simulink model "adip_saturation_sim"  (R2013a)
settings: Solver=ode4  StartTime=0.0  StopTime=10  FixedStep=0.001  RelTol=1e-3
values from neighbouring files (symbols this model uses):
  a1 = vertex(1,i)    [p2c13_ex5_adip_lqr_servo.m]    (also in p2c13_ex5_adip_oc_nominal_servo.m; p2c13_ex5_adip_oc_robust_servo.m)
  b1 = vertex(2,i)    [p2c13_ex5_adip_lqr_servo.m]    (also in p2c13_ex5_adip_oc_nominal_servo.m; p2c13_ex5_adip_oc_robust_servo.m)
  dtheta1_0 = 0    [p2c122_ex4_adip_oc_multiobjective_servo.m]    (also in p2c122_ex4_adip_oc_servo.m; p2c13_ex5_adip_lqr_servo.m; p2c13_ex5_adip_oc_nominal_servo.m; p2c13_ex5_adip_oc_robust_servo.m)
  dtheta2_0 = 0    [p2c122_ex4_adip_oc_multiobjective_servo.m]    (also in p2c122_ex4_adip_oc_servo.m; p2c13_ex5_adip_lqr_servo.m; p2c13_ex5_adip_oc_nominal_servo.m; p2c13_ex5_adip_oc_robust_servo.m)
  K = L*inv(X)    [p2c14_ex6_adip_oc_saturation.m]    (also in p2c15_ex7_adip_oc_gs_servo.m; p2c15_ex7_adip_oc_gs_servo_old.m)
  sat = sqrt(sigma2)    [p2c14_ex6_adip_oc_saturation.m]
  theta1_0 = 0    [p2c122_ex4_adip_oc_multiobjective_servo.m]    (also in p2c122_ex4_adip_oc_servo.m; p2c13_ex5_adip_lqr_servo.m; p2c13_ex5_adip_oc_nominal_servo.m; p2c13_ex5_adip_oc_robust_servo.m)
  theta2_0 = 0    [p2c122_ex4_adip_oc_multiobjective_servo.m]    (also in p2c122_ex4_adip_oc_servo.m; p2c13_ex5_adip_lqr_servo.m; p2c13_ex5_adip_oc_nominal_servo.m; p2c13_ex5_adip_oc_robust_servo.m)
undefined symbols (not defined in the file or in its folder): alpha2, alpha3, alpha5, mu2
settings Model: Creator=kawata  LastModifiedBy=kawata
settings DataIOCC: LimitDataPoints=off  SignalLoggingSaveFormat=ModelDataLogs
settings OptimizationCC: ExpressionDepthLimit=2147483647
settings DebuggingCC: FcnCallInpInsideContextMsg=UseLocalSettings
settings GRTTargetCC: CombineOutputUpdateFcns=off  GRTInterface=on

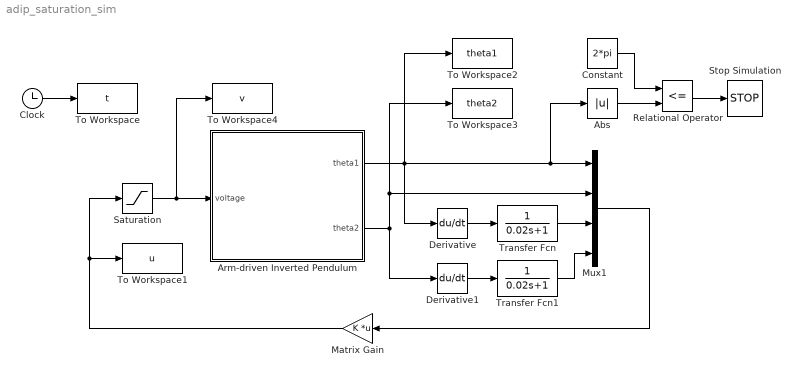
== system adip_saturation_sim ==
  Abs : Abs
  Arm-driven Inverted Pendulum : Subsystem
      mask Display: image(imread('adip.jpg'),'center')
  Clock : Clock
  Constant : Constant  Value=2*pi
  Derivative : Derivative
  Derivative1 : Derivative
  Matrix Gain : Gain  Gain=K  Multiplication=Matrix(K*u)  SaturateOnIntegerOverflow=on  OutDataTypeStr=Inherit: Same as input  ParamDataTypeStr=Inherit: Same as input
  Mux1 : Mux
  Relational Operator : RelationalOperator  Operator=<=  OutDataTypeStr=boolean
  Saturation : Saturate  UpperLimit=sat  LowerLimit=-sat
  Stop Simulation : Stop
  To Workspace : ToWorkspace  VariableName=t  SampleTime=-1
  To Workspace1 : ToWorkspace  VariableName=u  SampleTime=-1
  To Workspace2 : ToWorkspace  VariableName=theta1  SampleTime=-1
  To Workspace3 : ToWorkspace  VariableName=theta2  SampleTime=-1
  To Workspace4 : ToWorkspace  VariableName=v  SampleTime=-1
  Transfer Fcn : TransferFcn  Denominator=[0.02 1]
  Transfer Fcn1 : TransferFcn  Denominator=[0.02 1]
  wires:
  Clock/1 -> To Workspace/1
  Mux1/1 -> Matrix Gain/1
  Derivative/1 -> Transfer Fcn/1
  Transfer Fcn/1 -> Mux1/3
  Derivative1/1 -> Transfer Fcn1/1
  Transfer Fcn1/1 -> Mux1/4
  Arm-driven Inverted Pendulum/2(theta2) -> To Workspace3/1, Mux1/2, Derivative1/1
  Saturation/1 -> Arm-driven Inverted Pendulum/1(voltage), To Workspace4/1
  Matrix Gain/1 -> To Workspace1/1, Saturation/1
  Arm-driven Inverted Pendulum/1(theta1) -> To Workspace2/1, Abs/1, Mux1/1, Derivative/1
  Constant/1 -> Relational Operator/1
  Abs/1 -> Relational Operator/2
  Relational Operator/1 -> Stop Simulation/1

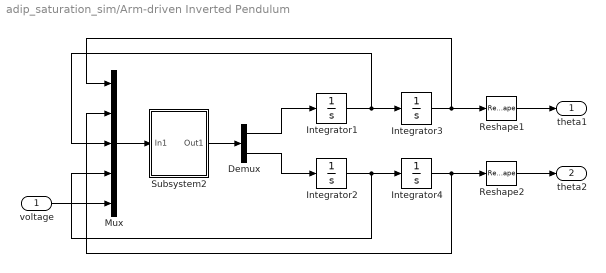
== system adip_saturation_sim/Arm-driven Inverted Pendulum ==
  voltage : Inport
  Demux : Demux  Outputs=2
  Integrator1 : Integrator  InitialCondition=dtheta1_0
  Integrator2 : Integrator  InitialCondition=dtheta2_0
  Integrator3 : Integrator  InitialCondition=theta1_0
  Integrator4 : Integrator  InitialCondition=theta2_0
  Mux : Mux  Inputs=5
  Reshape1 : Reshape
  Reshape2 : Reshape
  Subsystem2 : Subsystem
  theta1 : Outport
  theta2 : Outport  Port=2
  wires:
  voltage/1 -> Mux/5
  Integrator4/1 -> Mux/2, Reshape2/1
  Integrator3/1 -> Mux/1, Reshape1/1
  Integrator2/1 -> Integrator4/1, Mux/4
  Integrator1/1 -> Integrator3/1, Mux/3
  Demux/2 -> Integrator2/1
  Demux/1 -> Integrator1/1
  Mux/1 -> Subsystem2/1(In1)
  Subsystem2/1(Out1) -> Demux/1
  Reshape2/1 -> theta2/1
  Reshape1/1 -> theta1/1

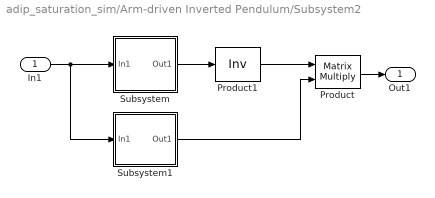
== system adip_saturation_sim/Arm-driven Inverted Pendulum/Subsystem2 ==
  In1 : Inport
  Product : Product  Multiplication=Matrix(*)  SaturateOnIntegerOverflow=on  InputSameDT=on  OutDataTypeStr=Inherit: Same as first input
  Product1 : Product  Inputs=/  Multiplication=Matrix(*)  SaturateOnIntegerOverflow=on  InputSameDT=on  OutDataTypeStr=Inherit: Same as first input
  Subsystem : Subsystem
  Subsystem1 : Subsystem
  Out1 : Outport
  wires:
  Subsystem/1(Out1) -> Product1/1
  Product1/1 -> Product/1
  Subsystem1/1(Out1) -> Product/2
  In1/1 -> Subsystem/1(In1), Subsystem1/1(In1)
  Product/1 -> Out1/1

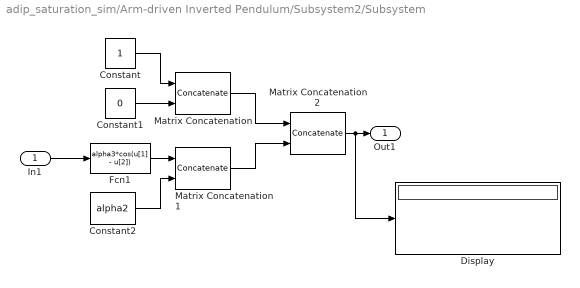
== system adip_saturation_sim/Arm-driven Inverted Pendulum/Subsystem2/Subsystem ==
  In1 : Inport
  Constant : Constant
  Constant1 : Constant  Value=0
  Constant2 : Constant  Value=alpha2
  Display : Display
  Fcn1 : Fcn  Expr=alpha3*cos(u[1] - u[2])
  Matrix Concatenation : Concatenate  Mode=Multidimensional array  ConcatenateDimension=2
  Matrix Concatenation1 : Concatenate  Mode=Multidimensional array  ConcatenateDimension=2
  Matrix Concatenation2 : Concatenate  Mode=Multidimensional array
  Out1 : Outport
  wires:
  Constant2/1 -> Matrix Concatenation1/2
  Fcn1/1 -> Matrix Concatenation1/1
  In1/1 -> Fcn1/1
  Matrix Concatenation/1 -> Matrix Concatenation2/1
  Matrix Concatenation1/1 -> Matrix Concatenation2/2
  Matrix Concatenation2/1 -> Display/1, Out1/1
  Constant/1 -> Matrix Concatenation/1
  Constant1/1 -> Matrix Concatenation/2

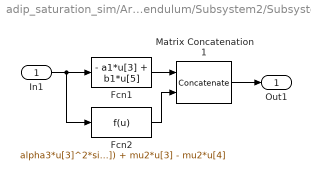
== system adip_saturation_sim/Arm-driven Inverted Pendulum/Subsystem2/Subsystem1 ==
  In1 : Inport
  Fcn1 : Fcn  Expr=- a1*u[3] + b1*u[5]
  Fcn2 : Fcn  Expr=alpha3*u[3]^2*sin(u[1] - u[2]) + alpha5*sin(u[2]) + mu2*u[3] - mu2*u[4]
  Matrix Concatenation1 : Concatenate  Mode=Multidimensional array
  Out1 : Outport
  wires:
  Fcn2/1 -> Matrix Concatenation1/2
  Fcn1/1 -> Matrix Concatenation1/1
  In1/1 -> Fcn2/1, Fcn1/1
  Matrix Concatenation1/1 -> Out1/1
